simulink model "problem6"  (R2020a)
settings: Solver=VariableStepAuto  StartTime=0.0  StopTime=10.0  RelTol=1e-3
settings Model: Creator=Jake  LastModifiedBy=Jake

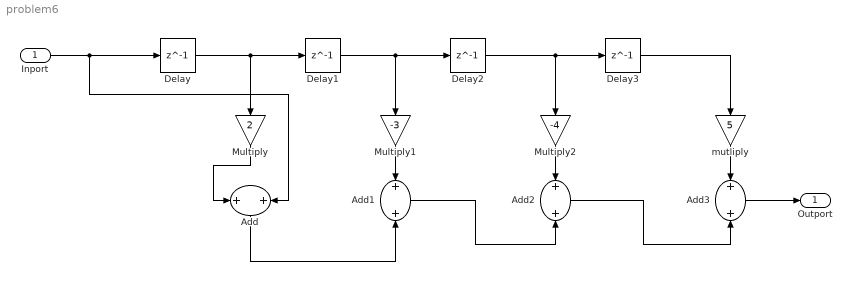
== system problem6 ==
  Inport : Inport
  Add{,1..3} (4 alike) : Sum
  Delay{,1..3} (4 alike) : Delay  DelayLength=1
  Multiply : Gain  Gain=2
  Multiply1 : Gain  Gain=-3
  Multiply2 : Gain  Gain=-4
  mutliply : Gain  Gain=5
  Outport : Outport
  wires:
  Inport/1 -> Add/2, Delay/1
  Delay/1 -> Multiply/1, Delay1/1
  Delay1/1 -> Multiply1/1, Delay2/1
  Delay2/1 -> Delay3/1, Multiply2/1
  Delay3/1 -> mutliply/1
  Multiply/1 -> Add/1
  Multiply1/1 -> Add1/1
  Add/1 -> Add1/2
  Multiply2/1 -> Add2/1
  Add1/1 -> Add2/2
  mutliply/1 -> Add3/1
  Add2/1 -> Add3/2
  Add3/1 -> Outport/1
